simulink model "sim07"  (R2012b)
settings: Solver=ode45  StartTime=0.0  StopTime=20  MaxStep=0.1  RelTol=1e-3
undefined symbols (not defined in the file): magnitude
libraries: simulink x1
settings Model: Creator=Administrator  LastModifiedBy=Administrator

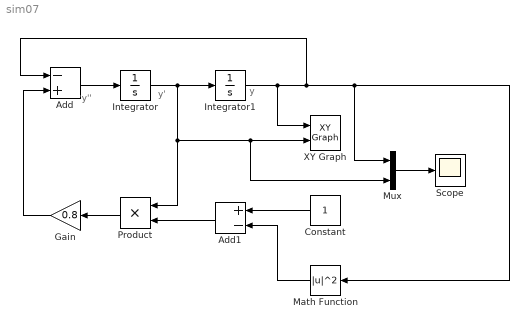
== system sim07 ==
  note: y
  note: y'
  note: y''
  Add : Sum  Inputs=-+
  Add1 : Sum  Inputs=+-
  Constant : Constant
  Gain : Gain  Gain=0.8
  Integrator : Integrator  InitialCondition=-2
  Integrator1 : Integrator  InitialCondition=4
  Math Function : Math  Operator=magnitude^2  SaturateOnIntegerOverflow=on
  Mux : Mux  Inputs=2
  Product : Product  RndMeth=Zero
  Scope : Scope
  XY Graph : simulink/Sinks/XY Graph  xmin=-5  xmax=5  ymin=-3  ymax=3  st=-1
  wires:
  Add/1 -> Integrator/1
  Integrator/1 -> Product/1, Mux/2, XY Graph/2, Integrator1/1
  Mux/1 -> Scope/1
  Constant/1 -> Add1/1
  Math Function/1 -> Add1/2
  Add1/1 -> Product/2
  Product/1 -> Gain/1
  Gain/1 -> Add/2
  Integrator1/1 -> XY Graph/1, Add/1, Mux/1, Math Function/1
